simulink model "TestDrive"  (R2019b)
settings: Solver=ode5  StartTime=0.0  StopTime=inf  FixedStep=0.01  RelTol=1e-3  EnableMultiTasking=on
values from neighbouring files (symbols this model uses):
  angle1 = [0 0 0 0 0 0 0 0 0 0 0 0 ... (12489 elements, 12489x1)]    [angle1.mat]
  indexswitch = 9635    [indexswitch.mat]
  speedref = 1    [speedref.mat]
  x_p = [21.5736 21.5810360806 21.5884855047 21.5959481254 21.6034237957 21.6109123686 21.618413697 21.6259276341 21.6334540327 21.6409927459 21.6485436267 21.6561065281 ... (12489 elements, 12489x1)]    [x_p.mat]
  x_p1 = [0 0 0 0 0 0 0 0 0 0 0 0 ... (12489 elements, 12489x1)]    [x_p1.mat]
  y_p = [6.59 6.59668187885 6.60334875784 6.61000077739 6.6166380779 6.62326079978 6.62986908343 6.63646306928 6.64304289772 6.64960870916 6.65616064401 6.66269884269 ... (12489 elements, 12489x1)]    [y_p.mat]
  y_p1 = [0 0 0 0 0 0 0 0 0 0 0 0 ... (12489 elements, 12489x1)]    [y_p1.mat]
libraries: simulink x2
settings Model: SimulationMode=accelerator  EnablePacing=on  Creator=20184717  LastModifiedBy=s161230
settings SolverCC: ConcurrentTasks=on  AutoInsertRateTranBlk=on  InsertRTBMode=Never (minimum delay)
settings DataIOCC: SaveFormat=StructureWithTime  ReturnWorkspaceOutputs=off
settings OptimizationCC: BlockReduction=off  OptimizeBlockIOStorage=off  BufferReuse=off  GlobalBufferReuse=off  ExpressionFolding=off  LocalBlockOutputs=off  OptimizeDataStoreBuffers=off  BusAssignmentInplaceUpdate=off
settings DebuggingCC: ArithmeticOperatorsInVariantConditions=warning
settings HardwareCC: ProdBitPerPointer=32  ProdBitPerSizeT=32  ProdBitPerPtrDiffT=32  ProdLargestAtomicFloat=None  ProdWordSize=32  ProdLongLongMode=on  ProdHWDeviceType=Generic->32-bit x86 compatible
settings SFSimCC: CustomCodeUndefinedFunction=UseInterfaceOnly
settings RTWCC: Description=Generic Real-Time Target  RTWCompilerOptimization=on
settings CodeAppCC: MaxIdLength=95
settings GRTTargetCC: TargetLangStandard=C89/C90 (ANSI)

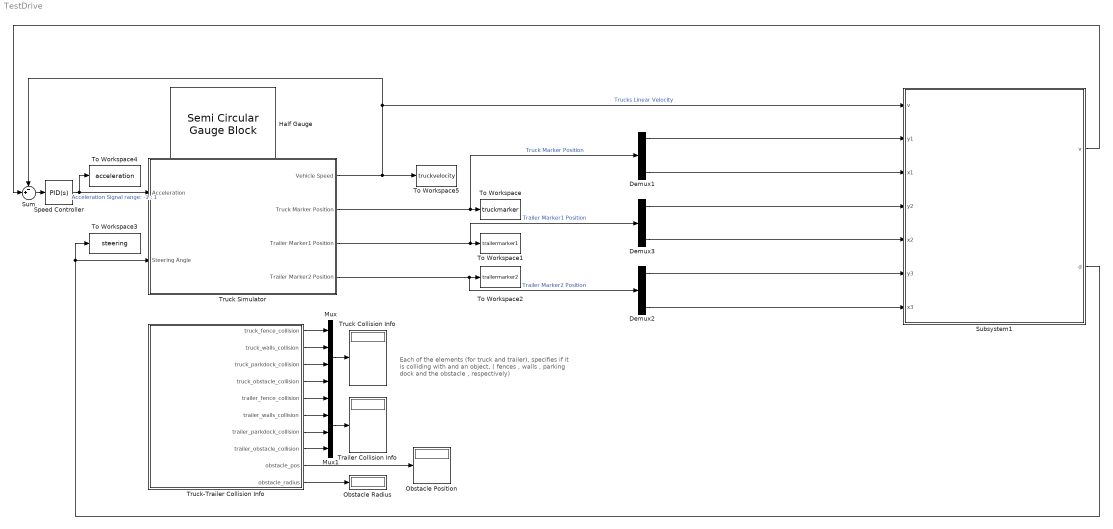
== system TestDrive ==
  note: Each of the elements (for truck and trailer),
      | specifies if it is colliding with and an object,
      | ( fences , walls , parking dock and the obstacle , respectively)
  Demux1 : Demux  Outputs=3
  Demux2 : Demux  Outputs=3
  Demux3 : Demux  Outputs=3
  Half Gauge : SemiCircularGaugeBlock  ScaleMax=5
  Mux : Mux
  Mux1 : Mux
  Obstacle Position : Display
  Obstacle Radius : Display
  Speed Controller : simulink/Continuous/PID Controller  Controller=PID  Form=Parallel  TimeDomain=Continuous-time  SampleTime=-1  IntegratorMethod=Forward Euler  FilterMethod=Forward Euler  ControllerParametersSource=internal  P=5  I=0.05  D=0  UseFilter=on  N=100  TunerSelectOption=Transfer Function Based (PID Tuner App)  InitialConditionSource=internal  InitialConditionForIntegrator=0  InitialConditionForFilter=0  DifferentiatorICPrevScaledInput=0  ExternalReset=none  TrackingMode=off  Kt=1  LimitOutput=on  UpperSaturationLimit=1  LowerSaturationLimit=-1  LinearizeAsGain=on  AntiWindupMode=none  Kb=1  POutMin=[]  POutMax=[]  IOutMin=[]  IOutMax=[]  DOutMin=[]  DOutMax=[]  NOutMin=[]  NOutMax=[]  SumOutMin=[]  SumOutMax=[]  SaturationOutMin=[]  SaturationOutMax=[]  PParamMin=[]  PParamMax=[]  IParamMin=[]  IParamMax=[]  DParamMin=[]  DParamMax=[]  NParamMin=[]  NParamMax=[]  KbParamMin=[]  KbParamMax=[]  KtParamMin=[]  KtParamMax=[]  KbOutMin=[]  KbOutMax=[]  KtOutMin=[]  KtOutMax=[]  IntegratorOutMin=[]  IntegratorOutMax=[]  FilterOutMin=[]  FilterOutMax=[]  SumI1OutMin=[]  SumI1OutMax=[]  SumI2OutMin=[]  SumI2OutMax=[]  SumI3OutMin=[]  SumI3OutMax=[]  SumI4OutMin=[]  SumI4OutMax=[]  SumDOutMin=[]  SumDOutMax=[]  DifferentiatorOutMin=[]  DifferentiatorOutMax=[]  FilterDiffOutCoefMin=[]  FilterDiffOutCoefMax=[]  ReciprocalOutMin=[]  ReciprocalOutMax=[]  SumDenOutMin=[]  SumDenOutMax=[]  SumNumOutMin=[]  SumNumOutMax=[]  DivideOutMin=[]  DivideOutMax=[]  IntegratorContinuousStateAttributes=''  IntegratorStateMustResolveToSignalObject=off  IntegratorRTWStateStorageClass=Auto  FilterContinuousStateAttributes=''  FilterStateMustResolveToSignalObject=off  FilterRTWStateStorageClass=Auto  ParallelPVariant=InternalParameters  IdealPVariant=Disabled  IVariant=InternalParameters  DVariant=InternalParameters  IntegratorVariant=Continuous  SatVariant=Enabled  AWVariant=Passthrough  PCopyVariant=Disabled  TRVariant=Disabled  FdbkBlocksVariant=Forward  IdealPFdbkVariant=Disabled  SatFdbkVariant=Disabled  DerivativeFilterVariant=ContFilter  NVariant=InternalParameters  NCopyVariant=Disabled  FilterICVariant=InternalICsFilter  IntegratorICVariant=InternalICs  ExternalResetVariant=Disabled  TRSumVariant=Passthrough  SumFdbkVariant=Disabled  SumVariant=Sum_PID
  Subsystem1 : Subsystem
  Sum : Sum  Inputs=-+|
  To Workspace : ToWorkspace  VariableName=truckmarker  SampleTime=-1
      settings: Save2DSignal=2-D array (concatenate along first dimension)
  To Workspace1 : ToWorkspace  VariableName=trailermarker1  SampleTime=-1
      settings: Save2DSignal=2-D array (concatenate along first dimension)
  To Workspace2 : ToWorkspace  VariableName=trailermarker2  SampleTime=-1
      settings: Save2DSignal=2-D array (concatenate along first dimension)
  To Workspace3 : ToWorkspace  VariableName=steering  SampleTime=-1
      settings: Save2DSignal=2-D array (concatenate along first dimension)
  To Workspace4 : ToWorkspace  VariableName=acceleration  SampleTime=-1
      settings: Save2DSignal=2-D array (concatenate along first dimension)
  To Workspace5 : ToWorkspace  VariableName=truckvelocity  SampleTime=-1
      settings: Save2DSignal=2-D array (concatenate along first dimension)
  Trailer Collision Info : Display
  Truck Collision Info : Display
  Truck Simulator : Subsystem
      mask DialogControl DescGroupVar Prompt: Truck Driver Block
      mask DialogControl DescTextVar Prompt: Interface for interacting with the simulated truck
      mask Display: image('icon.png')
  Truck-Trailer Collision Info : Subsystem
      mask Display: image('col_icon.png')
  wires:
  Truck Simulator/1(Vehicle Speed) -> Sum/1, Subsystem1/1("v "), To Workspace5/1  "Trucks Linear Velocity"
  Truck Simulator/2(Truck Marker Position) -> Demux1/1, To Workspace/1  "Truck Marker Position"
  Truck Simulator/3(Trailer Marker1 Position) -> Demux3/1, To Workspace1/1  "Trailer Marker1 Position"
  Truck Simulator/4(Trailer Marker2 Position) -> Demux2/1, To Workspace2/1  "Trailer Marker2 Position"
  Sum/1 -> Speed Controller/1
  Speed Controller/1 -> Truck Simulator/1(Acceleration), To Workspace4/1  "Acceleration Signal range: -1 : 1"
  Truck-Trailer Collision Info/1(truck_fence_collision) -> Mux/1
  Truck-Trailer Collision Info/2(truck_walls_collision) -> Mux/2
  Truck-Trailer Collision Info/3(truck_parkdock_collision) -> Mux/3
  Truck-Trailer Collision Info/4(truck_obstacle_collision) -> Mux/4
  Truck-Trailer Collision Info/5(trailer_fence_collision) -> Mux1/1
  Truck-Trailer Collision Info/6(trailer_walls_collision) -> Mux1/2
  Truck-Trailer Collision Info/7(trailer_parkdock_collision) -> Mux1/3
  Truck-Trailer Collision Info/8(trailer_obstacle_collision) -> Mux1/4
  Mux1/1 -> Trailer Collision Info/1
  Mux/1 -> Truck Collision Info/1
  Truck-Trailer Collision Info/9(obstacle_pos) -> Obstacle Position/1
  Truck-Trailer Collision Info/10(obstacle_radius) -> Obstacle Radius/1
  Subsystem1/2(d) -> To Workspace3/1, Truck Simulator/2(Steering Angle)
  Demux2/1 -> Subsystem1/6(y3)
  Demux2/3 -> Subsystem1/7("x3 ")
  Subsystem1/1(v) -> Sum/2
  Demux3/1 -> Subsystem1/4(y2)
  Demux3/3 -> Subsystem1/5(x2)
  Demux1/1 -> Subsystem1/2(y1)
  Demux1/3 -> Subsystem1/3(x1)

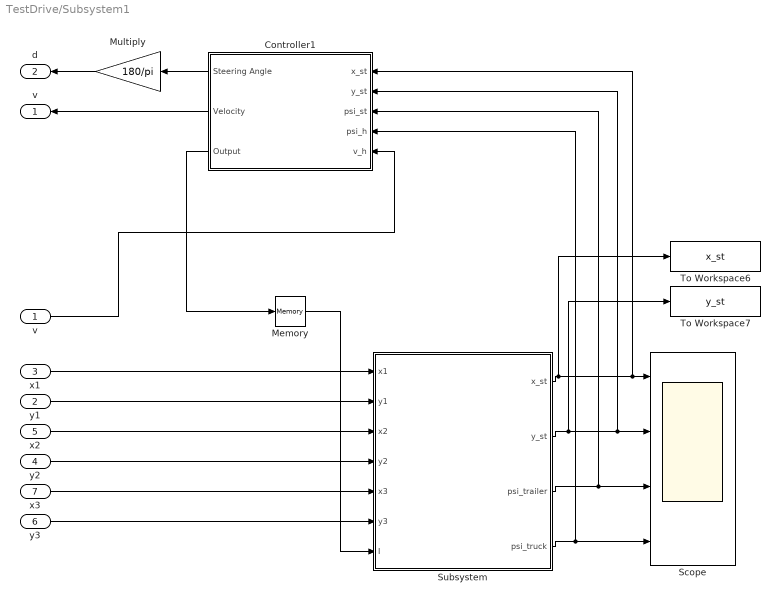
== system TestDrive/Subsystem1 ==
  "v " : Inport
  y1 : Inport  Port=2
  x1 : Inport  Port=3
  y2 : Inport  Port=4
  x2 : Inport  Port=5
  y3 : Inport  Port=6
  "x3 " : Inport  Port=7
  Controller1 : Subsystem
  Memory : Memory
  Multiply : Gain  Gain=180/pi
  Scope : Scope  NumInputPorts=4
  Subsystem : Subsystem
  To Workspace6 : ToWorkspace  VariableName=x_st  SampleTime=-1
  To Workspace7 : ToWorkspace  VariableName=y_st  SampleTime=-1
  v : Outport
  d : Outport  Port=2
  wires:
  Subsystem/1("x_st ") -> To Workspace6/1, Controller1/1(x_st), Scope/1
  "v "/1 -> Controller1/5(v_h)
  Subsystem/3("psi_trailer ") -> Controller1/3(psi_st), Scope/3
  Subsystem/4("psi_truck ") -> Controller1/4(psi_h), Scope/4
  Memory/1 -> Subsystem/7("I ")
  Subsystem/2(y_st) -> To Workspace7/1, Controller1/2(y_st), Scope/2
  Controller1/3(Output) -> Memory/1
  Controller1/1(Steering Angle) -> Multiply/1
  y2/1 -> Subsystem/4(y2)
  x1/1 -> Subsystem/1("x1 ")
  "x3 "/1 -> Subsystem/5("x3 ")
  x2/1 -> Subsystem/3(x2)
  Controller1/2("Velocity ") -> v/1
  y1/1 -> Subsystem/2(y1)
  Multiply/1 -> d/1
  y3/1 -> Subsystem/6(y3)

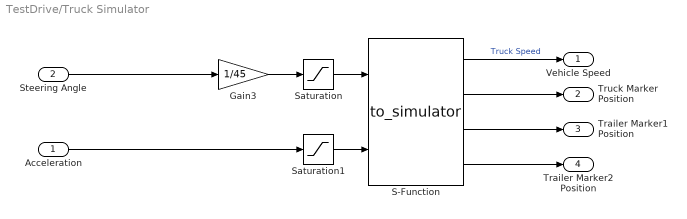
== system TestDrive/Truck Simulator ==
  Acceleration : Inport
  Steering Angle : Inport  Port=2
  Gain3 : Gain  Gain=1/45
  S-Function : S-Function  FunctionName=to_simulator  SFunctionDeploymentMode=off  EnableBusSupport=off
  Saturation : Saturate  UpperLimit=1  LowerLimit=-1
  Saturation1 : Saturate  UpperLimit=1  LowerLimit=-1
  Vehicle Speed : Outport  VectorParamsAs1DForOutWhenUnconnected=off
  Truck Marker Position : Outport  Port=2  VectorParamsAs1DForOutWhenUnconnected=off
  Trailer Marker1 Position : Outport  Port=3  VectorParamsAs1DForOutWhenUnconnected=off
  Trailer Marker2 Position : Outport  Port=4  VectorParamsAs1DForOutWhenUnconnected=off
  wires:
  S-Function/4 -> Trailer Marker2 Position/1
  Saturation/1 -> S-Function/1
  Gain3/1 -> Saturation/1
  Steering Angle/1 -> Gain3/1
  S-Function/3 -> Trailer Marker1 Position/1
  S-Function/2 -> Truck Marker Position/1
  Acceleration/1 -> Saturation1/1
  S-Function/1 -> Vehicle Speed/1  "Truck Speed"
  Saturation1/1 -> S-Function/2

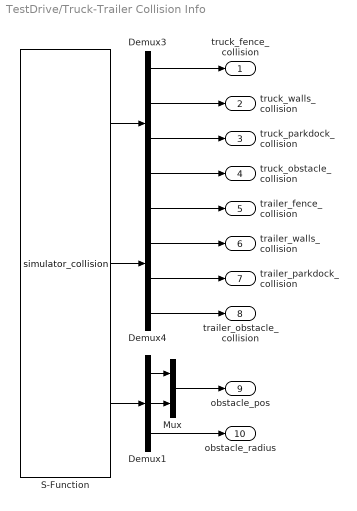
== system TestDrive/Truck-Trailer Collision Info ==
  Demux1 : Demux  Outputs=3
  Demux3 : Demux
  Demux4 : Demux
  Mux : Mux  Inputs=2
  S-Function : S-Function  FunctionName=simulator_collision  SFunctionDeploymentMode=off  EnableBusSupport=off
  truck_fence_collision : Outport  VectorParamsAs1DForOutWhenUnconnected=off
  truck_walls_collision : Outport  Port=2  VectorParamsAs1DForOutWhenUnconnected=off
  truck_parkdock_collision : Outport  Port=3  VectorParamsAs1DForOutWhenUnconnected=off
  truck_obstacle_collision : Outport  Port=4  VectorParamsAs1DForOutWhenUnconnected=off
  trailer_fence_collision : Outport  Port=5  VectorParamsAs1DForOutWhenUnconnected=off
  trailer_walls_collision : Outport  Port=6  VectorParamsAs1DForOutWhenUnconnected=off
  trailer_parkdock_collision : Outport  Port=7  VectorParamsAs1DForOutWhenUnconnected=off
  trailer_obstacle_collision : Outport  Port=8  VectorParamsAs1DForOutWhenUnconnected=off
  obstacle_pos : Outport  Port=9  VectorParamsAs1DForOutWhenUnconnected=off
  obstacle_radius : Outport  Port=10  VectorParamsAs1DForOutWhenUnconnected=off
  wires:
  Demux4/4 -> trailer_obstacle_collision/1
  Demux3/2 -> truck_walls_collision/1
  S-Function/2 -> Demux4/1
  Demux4/1 -> trailer_fence_collision/1
  Demux4/2 -> trailer_walls_collision/1
  Demux3/3 -> truck_parkdock_collision/1
  S-Function/1 -> Demux3/1
  Demux3/4 -> truck_obstacle_collision/1
  Demux3/1 -> truck_fence_collision/1
  Demux4/3 -> trailer_parkdock_collision/1
  S-Function/3 -> Demux1/1
  Demux1/3 -> obstacle_radius/1
  Demux1/1 -> Mux/1
  Demux1/2 -> Mux/2
  Mux/1 -> obstacle_pos/1

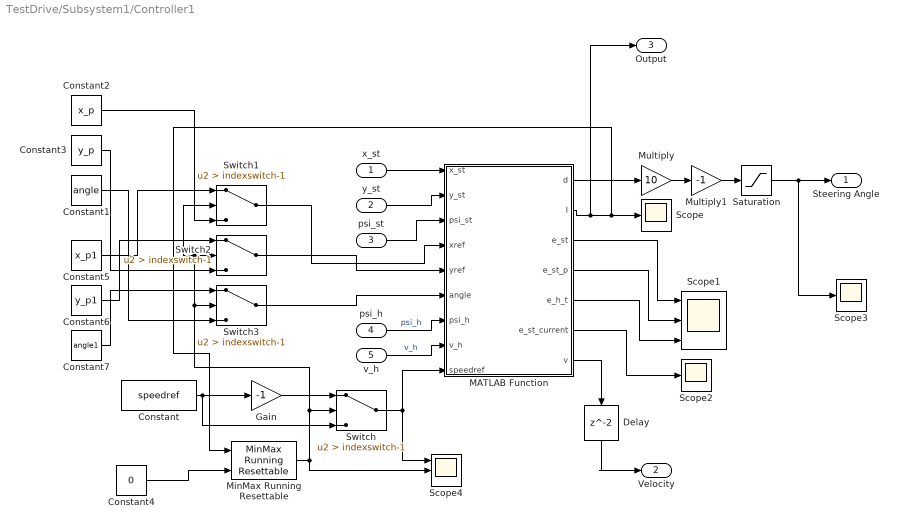
== system TestDrive/Subsystem1/Controller1 ==
  x_st : Inport  OutDataTypeStr=double
  y_st : Inport  Port=2  OutDataTypeStr=double
  psi_st : Inport  Port=3  OutDataTypeStr=double
  psi_h : Inport  Port=4  OutDataTypeStr=double
  v_h : Inport  Port=5  OutDataTypeStr=double
  Constant : Constant  Value=speedref
  Constant1 : Constant  Value=angle
  Constant2 : Constant  Value=x_p
  Constant3 : Constant  Value=y_p
  Constant4 : Constant  Value=0
  Constant5 : Constant  Value=x_p1
  Constant6 : Constant  Value=y_p1
  Constant7 : Constant  Value=angle1
  Delay : Delay  InitialCondition=1.0
  Gain : Gain  Gain=-1
  MATLAB Function : MATLAB Function  TreatAsAtomicUnit=on
  MinMax Running Resettable : simulink/Math Operations/MinMax Running Resettable  Function=max  vinit=0.0
  Multiply : Gain  Gain=10
  Multiply1 : Gain  Gain=-1
  Saturation : Saturate  UpperLimit=45/180*pi  LowerLimit=-45/180*pi  ZeroCross=off
  Scope : Scope
  Scope1 : Scope  NumInputPorts=3
  Scope2 : Scope
  Scope3 : Scope
  Scope4 : Scope  NumInputPorts=3
  Switch{,1..3} (4 alike) : Switch  Criteria=u2 > Threshold  Threshold=indexswitch-1
  Steering Angle : Outport  OutDataTypeStr=double
  "Velocity " : Outport  Port=2
  Output : Outport  Port=3
  wires:
  MATLAB Function/1(d) -> Multiply/1
  psi_st/1 -> MATLAB Function/3(psi_st)
  x_st/1 -> MATLAB Function/1(x_st)
  y_st/1 -> MATLAB Function/2(y_st)
  psi_h/1 -> MATLAB Function/7(psi_h)  "psi_h"
  v_h/1 -> MATLAB Function/8(v_h)  "v_h"
  Multiply/1 -> Multiply1/1
  MATLAB Function/2(I) -> Output/1, MinMax Running Resettable/1, Scope/1
  MATLAB Function/3(e_st) -> Scope1/1
  MATLAB Function/4(e_st_p) -> Scope1/2
  MATLAB Function/5(e_h_t) -> Scope1/3
  Saturation/1 -> Scope3/1, Steering Angle/1
  MATLAB Function/6(e_st_current) -> Scope2/1
  MATLAB Function/7(v) -> Delay/1
  Delay/1 -> "Velocity "/1
  Multiply1/1 -> Saturation/1
  Switch/1 -> Scope4/1, MATLAB Function/9(speedref)
  Constant/1 -> Switch/3, Gain/1
  Gain/1 -> Switch/1
  MinMax Running Resettable/1 -> Scope4/2, Switch2/2, Switch1/2, Switch3/2, Switch/2
  Constant4/1 -> MinMax Running Resettable/2
  Switch3/1 -> MATLAB Function/6(angle)
  Switch2/1 -> MATLAB Function/5(yref)
  Switch1/1 -> MATLAB Function/4(xref)
  Constant5/1 -> Switch1/1
  Constant2/1 -> Switch1/3
  Constant6/1 -> Switch2/1
  Constant7/1 -> Switch3/1
  Constant1/1 -> Switch3/3
  Constant3/1 -> Switch2/3

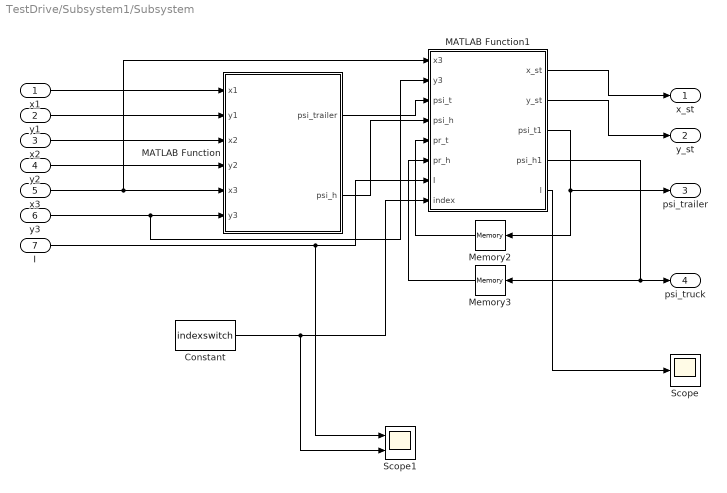
== system TestDrive/Subsystem1/Subsystem ==
  "x1 " : Inport
  y1 : Inport  Port=2
  x2 : Inport  Port=3
  y2 : Inport  Port=4
  "x3 " : Inport  Port=5
  y3 : Inport  Port=6
  "I " : Inport  Port=7
  Constant : Constant  Value=indexswitch
  MATLAB Function : MATLAB Function  TreatAsAtomicUnit=on
  MATLAB Function1 : MATLAB Function  TreatAsAtomicUnit=on
  Memory2 : Memory  InitialCondition=1.5902  InheritSampleTime=on
  Memory3 : Memory  InitialCondition=1.5902  InheritSampleTime=on
  Scope : Scope
  Scope1 : Scope  NumInputPorts=2
  "x_st " : Outport
  y_st : Outport  Port=2
  "psi_trailer " : Outport  Port=3
  "psi_truck " : Outport  Port=4
  wires:
  Memory3/1 -> MATLAB Function1/6(pr_h)
  MATLAB Function/2(psi_h) -> MATLAB Function1/4(psi_h)
  MATLAB Function1/4(psi_h1) -> "psi_truck "/1, Memory3/1
  MATLAB Function1/3(psi_t1) -> Memory2/1, "psi_trailer "/1
  Memory2/1 -> MATLAB Function1/5(pr_t)
  MATLAB Function/1(psi_trailer) -> MATLAB Function1/3(psi_t)
  "x1 "/1 -> MATLAB Function/1(x1)
  y1/1 -> MATLAB Function/2(y1)
  x2/1 -> MATLAB Function/3(x2)
  "x3 "/1 -> MATLAB Function1/1(x3), MATLAB Function/5(x3)
  y2/1 -> MATLAB Function/4(y2)
  y3/1 -> MATLAB Function1/2(y3), MATLAB Function/6(y3)
  MATLAB Function1/1(x_st) -> "x_st "/1
  MATLAB Function1/2(y_st) -> y_st/1
  "I "/1 -> Scope1/1, MATLAB Function1/7(I)
  Constant/1 -> Scope1/2, MATLAB Function1/8(index)
  MATLAB Function1/5(l) -> Scope/1

== matlab function TestDrive/Subsystem1/Subsystem/MATLAB Function1 ==
  data: x3 input; y3 input; x_st output; y_st output; psi_t input; psi_t1 output; psi_h input; pr_t input; pr_h input; psi_h1 output; I input; index input; l output
function [x_st, y_st, psi_t1, psi_h1, l] = fcn(x3, y3, psi_t, psi_h, pr_t, pr_h, I, index)
% l = 3.025;
if I<1200
    l = 1.025;
else if I<index
l = 1.025;
else
    l = 3.025;
    end
end

P1 = [pr_t psi_t];
Q1 = unwrap(P1);

P2 = [pr_h psi_h];
Q2 = unwrap(P2);

psi_t1 = Q1(2);
psi_h1 = Q2(2);

x3n = abs(x3-39);
y3n = y3+25.8;

x_stn = x3n-cos(psi_t1)*l;
y_stn = y3n-sin(psi_t1)*l;

x_st = x_stn;
y_st = y_stn;

== matlab function TestDrive/Subsystem1/Subsystem/MATLAB Function ==
  data: x1 input; y1 input; x2 input; y2 input; x3 input; y3 input; psi_trailer output; psi_h output
function [psi_trailer, psi_h] = fcn(x1, y1, x2, y2, x3, y3)
l = 3.025;

x1n = abs(x1-39);
y1n = y1+25.8;

x2n = abs(x2-39);
y2n = y2+25.8;

x3n = abs(x3-39);
y3n = y3+25.8;

angle_trailer = atan((y2n-y3n)/(x2n-x3n));
angle_head = atan((y1n-y2n)/(x1n-x2n));
psi_trailer = 0;
psi_h = 0;

if x2n>x3n && y2n>y3n || x2n>x3n && y2n<y3n
    psi_trailer = angle_trailer;
    psi_h = 0;
else if x2n<x3n && y2n>y3n || x2n<x3n && y2n<y3n
        psi_trailer = pi+angle_trailer;
        psi_h = 0;
    else if x2n==x3n
            if y2n>y3n
                psi_trailer = 0.5*pi;
                psi_h = 0;
            else
                psi_trailer = -0.5*pi;
                psi_h = 0;
            end
        else if y2n==y3n
                if x2n>x3n
                    psi_trailer = 0;
                    psi_h = 0;
                else
                    psi_trailer = -pi;
                    psi_h = 0;
                end
            end
            
        end
    end
end

if x1n>x2n && y1n>y2n || x1n>x2n && y1n<y2n
    psi_h = angle_head;
    psi_trailer = psi_trailer;
else if x1n<x2n && y1n>y2n || x1n<x2n && y1n<y2n
        psi_h = pi+angle_head;
        psi_trailer = psi_trailer;
        
    else if x1n==x2n
            if y1n>y2n
                psi_h = 0.5*pi;
                psi_trailer = psi_trailer;
                
            else
                psi_h = -0.5*pi;
                psi_trailer = psi_trailer;
                
            end
        else if y1n==y2n
                if x1n>x2n
                    psi_h = 0;
                    psi_trailer = psi_trailer;
                    
                else
                    psi_h = -pi;
                    psi_trailer = psi_trailer;
                    
                end
            end
            
        end
    end
end


% add conversion when y2=y3 and x2=x3
% normalize angle to between -2pi and 2pi


% x_st = 39-x_stn;
% y_st = y_stn-25.8;

== matlab function TestDrive/Subsystem1/Controller1/MATLAB Function ==
  data: d output; I output; x_st input; y_st input; psi_st input; xref input; yref input; angle input; psi_h input; v_h input; e_st output; e_st_p output; e_h_t output; e_st_current output; v output; speedref input
function [d, I, e_st, e_st_p, e_h_t, e_st_current, v]  = Error(x_st, y_st, psi_st, xref, yref, angle, psi_h,v_h,speedref)

if speedref == 1
    [~, I] = min(sqrt((xref-x_st).^2+(yref-y_st).^2));
    lookahead = 200;
    K1 = 80;%2
    K2 = 7.6;%13
    l_h = 0.22;
    l_st = 0.72;
%     l_h = 4.58;
%     l_st = 9.58;
    
    %1.0m
    lookahead = 77; %77
    K1 = 75;        %75
    K2 = 12;        %12
    
    %0.9m
    lookahead = 82;
    K1 = 76;
    K2 = 12;
    
    %0.8m
    lookahead = 86;
    K1 = 77;
    K2 = 12;
        
    %0.7m
    lookahead = 88;
    K1 = 79;
    K2 = 12;
    
    %0.6m
    lookahead = 95;
    K1 = 79;
    K2 = 12;
    
    %0.5m
    lookahead = 110;
    K1 = 79;
    K2 = 12;
    
    %0.4m
    lookahead = 500;
    K1 = 1.2;
    K2 = 1;
    
    %% final values forward controller
    lookahead = 200;
    K1 = 1.3; %max 1.3
    K2 = 3; %max 4.5
    
    lookahead = 200;
    K1 = .9; %max 1.3
    K2 = .9; %max 4.5
    
    lookahead = 200;
    K1 = .9; %max 1.3
    K2 = .9; %max 4.5
    
    %0.35m
%     lookahead = 210;
%     K1 = 86;
%     K2 = 12;
    
    %0.3m
%     lookahead = 220;
%     K1 = 90;
%     K2 = 12;
%     
    if I < length(angle) - 1
        stop = 0;
        
        if I < length(angle) - lookahead
            
             e_st_current = -sin(psi_st)*(x_st-xref(I))+cos(psi_st)*(y_st-yref(I));
             %define errors
%              e_st = -sin(psi_st)*(x_st-xref(I+lookahead))+cos(psi_st)*(y_st-yref(I+lookahead));
             e_st = -sin(psi_st)*(-x_st+xref(I+lookahead))+cos(psi_st)*(-y_st+yref(I+lookahead));

             e_st_p = psi_st - angle(I+lookahead);
             
             %difference heading truck and heading trailer
             e_h_t = psi_h-psi_st;
             
             %desired value for e_h_t (input u)
%              u = -atan((l_st/v_h)*(K1*e_st_p/cos(e_h_t)+e_st*v_h*sin(e_st_p)/e_st_p));
%              psi = -atan((l_st/(v_h))*(-K1*e_st_p/cos(e_h_t)-e_st*v_h*(sin(e_st_p)/e_st_p)));
             value = (l_st/v_h)*(-K1*e_st_p-e_st*v_h*sin(e_st_p)/e_st_p);
             if value > 1
                 value = 1;
             else if value < -1
                     value = -1;
                 else
                     value = value;
                 end
             end
             psi = -asin(value);

%              psi = -asin((l_st/v_h)*(-K1*e_st_p-e_st*v_h*sin(e_st_p)/e_st_p));
                                 
             %dynamics
             e_st_p_dot = v_h/l_st*sin(e_h_t);
%              e_st_dot = v_h*cos(e_h_t)*sin(e_st_p);
             e_st_dot = v_h*sin(e_st_p);
             
%              u_dot = -1*(1/(1+((l_st/v_h)*K1*e_st_p/cos(e_h_t)+e_st*v_h*sin(e_st_p)/e_st_p)^2))*(l_st/v_h)*(K1*e_st_p_dot/cos(e_h_t)+e_st_dot*v_h*sin(e_st_p)/e_st_p+e_st*v_h*e_st_p_dot*(cos(e_st_p)*e_st_p-sin(e_st_p))/(e_st_p^2));
             
%              x = (l_st/(v_h*cos(e_h_t)))*(-K1*e_st_p-e_st*v_h*(sin(e_st_p)/e_st_p));
             x = (l_st/v_h)*(-K1*e_st_p-e_st*v_h*sin(e_st_p)/e_st_p);
             x1_dot = e_st_p_dot*((e_st*sin(e_st_p)-e_st_p*e_st*cos(e_st_p))/(e_st_p^2)-(K1*l_st)/v_h)-(e_st_p*e_st_dot*sin(e_st_p))/(e_st_p^2);
             if (1-x^2)<0
                 x = 0.9999999;
             end
             psi_dot = (1/(sqrt(1-x^2)))*x1_dot;
             
%              x1_dot = (-v_h*l_st*K1*cos(e_h_t)*e_st_p_dot-v_h*l_st*K1*e_st_p*sin(e_h_t)*e_h_t_dot)/(v_h*v_h*cos(e_h_t)*cos(e_h_t)); 
%              x2_dot = (-e_st_p*l_st*tan(e_st_p)*e_st_dot-l_st*e_st*e_st_p_dot/(cos(e_st_p)^2)+l_st*e_st*tan(e_st_p)*e_st_p_dot)/(e_st_p^2);
%              psi_dot = -(1/(1+x^2))*(x1_dot+x2_dot);
             %difference between desired and actual
%              z = (psi_h-psi_st)-u;
%              z = e_h_t - psi;
             z = psi-e_h_t;
            
             
             %steering angle to achieve required path
%              d = asin((l_h/v_h)*(-K2*z+u_dot+(v_h/l_st)*sin(psi_h-psi_st)));
             value = (l_h/v_h)*(K2*z+psi_dot+(v_h/l_st)*sin(psi));
             if value > 1
                 value = 1;
             else if value < -1
                     value = -1;
                 else
                     value = value;
                 end
             end
             d = asin(value);
             %trying something
%              d = atan((l_h/v_h)*(-K2*u+v_h/l_st*tan(e_h_t)*cos(e_h_t)));
%              d = asin((l_h/v_h)*(K2*z+psi_dot+(v_h/l_st)*sin(psi)));
             if I < 2000
                 v = 1;
             else if I<2500
                     v=2;
                 else
             v = 3;
                 end
             end
        else
            %define erros
             e_st_current = -sin(psi_st)*(x_st-xref(I))+cos(psi_st)*(y_st-yref(I));
%              e_st = -sin(psi_st)*(x_st-xref(end))+cos(psi_st)*(y_st-yref(end));
             e_st = -sin(psi_st)*(-x_st+xref(end))+cos(psi_st)*(-y_st+yref(end));

             e_st_p = psi_st - angle(end);
             
             %difference heading truck and heading trailer
             e_h_t = psi_h-psi_st;
             
             %desired value for e_h_t (input u)
%              u = -atan((l_st/v_h)*(K1*e_st_p/cos(e_h_t)+e_st*v_h*sin(e_st_p)/e_st_p));
%              psi = -atan((l_st/(v_h))*(-K1*e_st_p/cos(e_h_t)-e_st*v_h*(sin(e_st_p)/e_st_p)));
             value = (l_st/v_h)*(-K1*e_st_p-e_st*v_h*sin(e_st_p)/e_st_p);
%              if value > 1
%                  value = 1;
%              else if value < -1
%                      value = -1;
%                  else
%                      value = value;
%                  end
%              end
             psi = -asin(value);
             %dynamics
             e_st_p_dot = v_h/l_st*sin(e_h_t);
             e_st_dot = v_h*cos(e_h_t)*sin(e_st_p);
%              u_dot = -1*(1/(1+((l_st/v_h)*K1*e_st_p/cos(e_h_t)+e_st*v_h*sin(e_st_p)/e_st_p)^2))*(l_st/v_h)*(K1*e_st_p_dot/cos(e_h_t)+e_st_dot*v_h*sin(e_st_p)/e_st_p+e_st*v_h*e_st_p_dot*(cos(e_st_p)*e_st_p-sin(e_st_p))/(e_st_p^2));
             x = (l_st/v_h)*(-K1*e_st_p-e_st*v_h*sin(e_st_p)/e_st_p);
             x1_dot = e_st_p_dot*((e_st*sin(e_st_p)-e_st_p*e_st*cos(e_st_p))/(e_st_p^2)-(K1*l_st)/v_h)-(e_st_p*e_st_dot*sin(e_st_p))/(e_st_p^2);
%              if (1-x^2)<0
%                  x = 0.9999999;
%              end
             
             psi_dot = (1/(sqrt(1-x^2)))*x1_dot;
%              x = (l_st/(v_h*cos(e_h_t)))*(-K1*e_st_p-e_st*v_h*(sin(e_st_p)/e_st_p));
%              
%              x1_dot = (-v_h*l_st*K1*cos(e_h_t)*e_st_p_dot-v_h*l_st*K1*e_st_p*sin(e_h_t)*e_h_t_dot)/(v_h*v_h*cos(e_h_t)*cos(e_h_t)); 
%              x2_dot = (-e_st_p*l_st*tan(e_st_p)*e_st_dot-l_st*e_st*e_st_p_dot/(cos(e_st_p)^2)+l_st*e_st*tan(e_st_p)*e_st_p_dot)/(e_st_p^2);
%              psi_dot = -(1/(1+x^2))*(x1_dot+x2_dot);
             %difference between desired and actual
%              z = (psi_h-psi_st)-u;
%              z =  e_h_t-psi;
             z=psi-e_h_t;
             %steering angle to achieve required path
%              d = asin((l_h/v_h)*(-K2*z+u_dot+(v_h/l_st)*sin(psi_h-psi_st)));
             value = (l_h/v_h)*(K2*z+psi_dot+(v_h/l_st)*sin(psi));
%              if value > 1
%                  value = 1;
%              else if value < -1
%                      value = -1;
%                  else
%                      value = value;
%                  end
%              end
             d = asin(value);
%              d = asin((l_h/v_h)*(K2*z+psi_dot+(v_h/l_st)*sin(psi)));
             v = 3;
        end
    else
        e_st_current = 0;
        e_st = 0;
        e_st_p = 0;
        e_h_t = 0;
        d = 0;
        v = 0;
    end
else
[~, I] = min(sqrt((xref-x_st).^2+(yref-y_st).^2));
    lookahead = 200;
    K1 = 80;%2
    K2 = 7.6;%13
    l_h = 0.22;
    l_st = 0.72;
    
    %1.0m
    lookahead = 77; %77
    K1 = 75;        %75
    K2 = 12;        %12
    
    %0.9m
    lookahead = 82;
    K1 = 76;
    K2 = 12;
    
    K1 = 65;
    K2 = 8;
    
%     %0.8m
%     lookahead = 86;
%     K1 = 77;
%     K2 = 12;
        
    %0.7m
%     lookahead = 88;
%     K1 = 79;
%     K2 = 12;
%     
%     0.6m
%     lookahead = 95;
%     K1 = 79;
%     K2 = 12;
%     
%     0.5m
    lookahead = 110;
    K1 = 79;
    K2 = 12;
%     
%     %0.4m
%     lookahead = 150;
%     K1 = 79;
%     K2 = 12;
    
    %0.35m
%     lookahead = 210;
%     K1 = 86;
%     K2 = 12;
    
    %0.3m
    lookahead = 60;
    K1 = 65;
    K2 = 7.5;
    
    lookahead = 40;
    K1 = 80;
    K2 = 8;
    
    lookahead = 1200;
    K1 =500;
    K2 =1;
    
    lookahead = 400;
    K1 =500;
    K2 =60;
    
    lookahead = 400;
    K1 = 35;
    K2 = 1;
    
    lookahead = 500;
    K1 = 55;
    K2 = 1;
    
    lookahead = 500;
    K1 = 55;
    K2 = 1.6;

if I < length(angle) - 1
        stop = 0;
        
        if I < length(angle) - lookahead
            
            %define errors
             e_st = -sin(psi_st)*(x_st-xref(I+lookahead))+cos(psi_st)*(y_st-yref(I+lookahead));
             e_st_p = psi_st - angle(I+lookahead);
             e_st_current = -sin(psi_st)*(x_st-xref(I))+cos(psi_st)*(y_st-yref(I));
             e_st = -sin(psi_st)*(-x_st+xref(I+lookahead))+cos(psi_st)*(-y_st+yref(I+lookahead));
             
             %difference heading truck and heading trailer
             e_h_t = psi_h-psi_st;
             
             %desired value for e_h_t (input u)
             u = -atan((l_st/v_h)*(K1*e_st_p/cos(e_h_t)+e_st*v_h*sin(e_st_p)/e_st_p));
             
             %dynamics
             e_st_p_dot = v_h/l_st*sin(e_h_t);
             e_st_dot = v_h*cos(e_h_t)*sin(e_st_p);
             u_dot = -1*(1/(1+((l_st/v_h)*K1*e_st_p/cos(e_h_t)+e_st*v_h*sin(e_st_p)/e_st_p)^2))*(l_st/v_h)*(K1*e_st_p_dot/cos(e_h_t)+e_st_dot*v_h*sin(e_st_p)/e_st_p+e_st*v_h*e_st_p_dot*(cos(e_st_p)*e_st_p-sin(e_st_p))/(e_st_p^2));
    
             %difference between desired and actual
             z = (psi_h-psi_st)-u;
             
             %steering angle to achieve required path
             value = (l_h/v_h)*(-K2*z+u_dot+(v_h/l_st)*sin(psi_h-psi_st));
             if value < -1
                 value = -1;
             else if value > 1
                     value = 1;
                 else 
                     value = value;
                 end
             end
             d = asin(value);
             %trying something
%              d = atan((l_h/v_h)*(-K2*u+v_h/l_st*tan(e_h_t)*cos(e_h_t)));
             v=-1.5;
        else
            %define erros
             e_st = -sin(psi_st)*(x_st-xref(end))+cos(psi_st)*(y_st-yref(end));
             e_st_p = psi_st - angle(end);
             e_st_current = -sin(psi_st)*(x_st-xref(I))+cos(psi_st)*(y_st-yref(I));
             e_st = -sin(psi_st)*(-x_st+xref(end))+cos(psi_st)*(-y_st+yref(end));
             %difference heading truck and heading trailer
             e_h_t = psi_h-psi_st;
             
             %desired value for e_h_t (input u)
             u = -atan((l_st/v_h)*(K1*e_st_p/cos(e_h_t)+e_st*v_h*sin(e_st_p)/e_st_p));
             
             %dynamics
             e_st_p_dot = v_h/l_st*sin(e_h_t);
             e_st_dot = v_h*cos(e_h_t)*sin(e_st_p);
             u_dot = -1*(1/(1+((l_st/v_h)*K1*e_st_p/cos(e_h_t)+e_st*v_h*sin(e_st_p)/e_st_p)^2))*(l_st/v_h)*(K1*e_st_p_dot/cos(e_h_t)+e_st_dot*v_h*sin(e_st_p)/e_st_p+e_st*v_h*e_st_p_dot*(cos(e_st_p)*e_st_p-sin(e_st_p))/(e_st_p^2));
             
             %difference between desired and actual
             z = (psi_h-psi_st)-u;
             
             %steering angle to achieve required path
             value = (l_h/v_h)*(-K2*z+u_dot+(v_h/l_st)*sin(psi_h-psi_st));
             if value < -1
                 value = -1;
             else if value > 1
                     value = 1;
                 else 
                     value = value;
                 end
             end
             d = asin(value);
             v = -0.5;
        end
    else
        e_st_current = 0;
        e_st = 0;
        e_st_p = 0;
        e_h_t = 0;
        d = 0;
        stop = 1;
        v = 0;
    end
end
